simulink model "filtros2"  (R2018b)
settings: Solver=VariableStepAuto  StartTime=0.0  StopTime=10.0  RelTol=1e-3
settings Model: Creator=vini  LastModifiedBy=vini

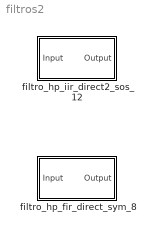
== system filtros2 ==
  filtro_hp_fir_direct_sym_8 : Subsystem  Tag=FilterWizardSubSystem
      settings: ErrorFcn=dspFilterRealizedInBasicElemsAlgLoopErrFcnCallback
  filtro_hp_iir_direct2_sos_12 : Subsystem  Tag=FilterWizardSubSystem
      settings: ErrorFcn=dspFilterRealizedInBasicElemsAlgLoopErrFcnCallback

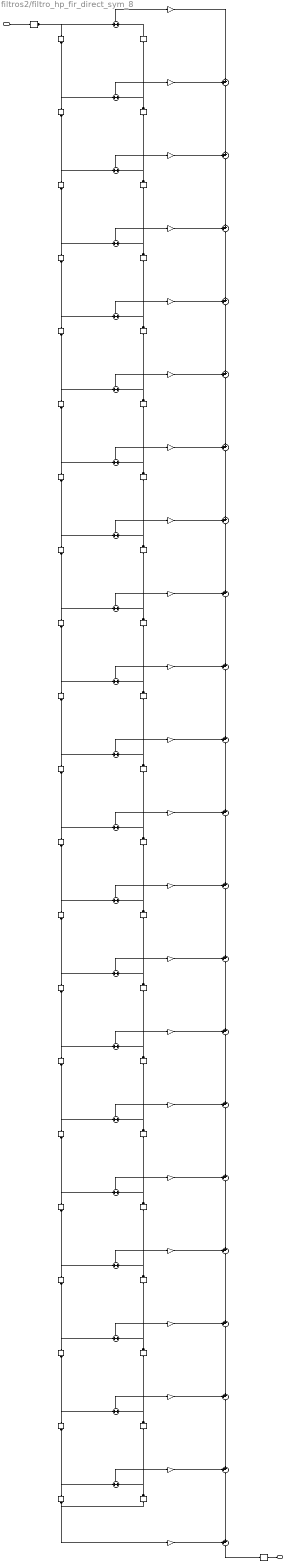
== system filtros2/filtro_hp_fir_direct_sym_8 ==
  Input : Inport
  BodyDelayL{2..21} (20 alike) : Delay  DelayLength=1  InitialCondition=0  InputProcessing=Columns as channels (frame based)
  BodyDelayR{2..21} (20 alike) : Delay  DelayLength=1  InitialCondition=0  InputProcessing=Columns as channels (frame based)
  BodySumL{2..21} (20 alike) : Sum  Inputs=+|+  AccumDataTypeStr=fixdt(1,17,15)  OutDataTypeStr=fixdt(1,17,15)  RndMeth=Convergent
  BodySumR{2..21} (20 alike) : Sum  Inputs=++|  AccumDataTypeStr=fixdt(1,25,23)  OutDataTypeStr=fixdt(1,25,23)  RndMeth=Convergent
  ConvertIn : DataTypeConversion  OutDataTypeStr=fixdt(1,16,15)  RndMeth=Nearest  SaturateOnIntegerOverflow=on
  ConvertOut : DataTypeConversion  OutDataTypeStr=fixdt(1,25,23)  RndMeth=Convergent
  FootDelayL22 : Delay  DelayLength=1  InitialCondition=0  InputProcessing=Columns as channels (frame based)
  FootSumR22 : Sum  Inputs=++|  AccumDataTypeStr=fixdt(1,25,23)  OutDataTypeStr=fixdt(1,25,23)  RndMeth=Convergent
  HeadDelayR1 : Delay  DelayLength=1  InitialCondition=0  InputProcessing=Columns as channels (frame based)
  HeadSumL1 : Sum  Inputs=+|+  AccumDataTypeStr=fixdt(1,17,15)  OutDataTypeStr=fixdt(1,17,15)  RndMeth=Convergent
  h(1) : Gain  Gain=-0.00532709506172761044  ParamDataTypeStr=fixdt(1,8,8)  OutDataTypeStr=fixdt(1,24,23)  RndMeth=Convergent
  h(10) : Gain  Gain=0.00894421000991611065  ParamDataTypeStr=fixdt(1,8,8)  OutDataTypeStr=fixdt(1,24,23)  RndMeth=Convergent
  h(11) : Gain  Gain=-0.0216421575545340458  ParamDataTypeStr=fixdt(1,8,8)  OutDataTypeStr=fixdt(1,24,23)  RndMeth=Convergent
  h(12) : Gain  Gain=0.0030362156599829525  ParamDataTypeStr=fixdt(1,8,8)  OutDataTypeStr=fixdt(1,24,23)  RndMeth=Convergent
  h(13) : Gain  Gain=0.0265962407774834042  ParamDataTypeStr=fixdt(1,8,8)  OutDataTypeStr=fixdt(1,24,23)  RndMeth=Convergent
  h(14) : Gain  Gain=-0.0224925554974460436  ParamDataTypeStr=fixdt(1,8,8)  OutDataTypeStr=fixdt(1,24,23)  RndMeth=Convergent
  h(15) : Gain  Gain=-0.0206671663559229203  ParamDataTypeStr=fixdt(1,8,8)  OutDataTypeStr=fixdt(1,24,23)  RndMeth=Convergent
  h(16) : Gain  Gain=0.0463858207415749138  ParamDataTypeStr=fixdt(1,8,8)  OutDataTypeStr=fixdt(1,24,23)  RndMeth=Convergent
  h(17) : Gain  Gain=-0.00352514866909382297  ParamDataTypeStr=fixdt(1,8,8)  OutDataTypeStr=fixdt(1,24,23)  RndMeth=Convergent
  h(18) : Gain  Gain=-0.0696283973383888116  ParamDataTypeStr=fixdt(1,8,8)  OutDataTypeStr=fixdt(1,24,23)  RndMeth=Convergent
  h(19) : Gain  Gain=0.0620411228742990054  ParamDataTypeStr=fixdt(1,8,8)  OutDataTypeStr=fixdt(1,24,23)  RndMeth=Convergent
  h(2) : Gain  Gain=0.00150016559407488014  ParamDataTypeStr=fixdt(1,8,8)  OutDataTypeStr=fixdt(1,24,23)  RndMeth=Convergent
  h(20) : Gain  Gain=0.0865544797646948944  ParamDataTypeStr=fixdt(1,8,8)  OutDataTypeStr=fixdt(1,24,23)  RndMeth=Convergent
  h(21) : Gain  Gain=-0.292552788167892264  ParamDataTypeStr=fixdt(1,8,8)  OutDataTypeStr=fixdt(1,24,23)  RndMeth=Convergent
  h(22) : Gain  Gain=0.389496680318399457  ParamDataTypeStr=fixdt(1,8,8)  OutDataTypeStr=fixdt(1,24,23)  RndMeth=Convergent
  h(3) : Gain  Gain=0.00628495279823278012  ParamDataTypeStr=fixdt(1,8,8)  OutDataTypeStr=fixdt(1,24,23)  RndMeth=Convergent
  h(4) : Gain  Gain=-0.00636828988327803585  ParamDataTypeStr=fixdt(1,8,8)  OutDataTypeStr=fixdt(1,24,23)  RndMeth=Convergent
  h(5) : Gain  Gain=-0.00403452349221034706  ParamDataTypeStr=fixdt(1,8,8)  OutDataTypeStr=fixdt(1,24,23)  RndMeth=Convergent
  h(6) : Gain  Gain=0.0111906482400220622  ParamDataTypeStr=fixdt(1,8,8)  OutDataTypeStr=fixdt(1,24,23)  RndMeth=Convergent
  h(7) : Gain  Gain=-0.00231967061384724497  ParamDataTypeStr=fixdt(1,8,8)  OutDataTypeStr=fixdt(1,24,23)  RndMeth=Convergent
  h(8) : Gain  Gain=-0.0130613282623932899  ParamDataTypeStr=fixdt(1,8,8)  OutDataTypeStr=fixdt(1,24,23)  RndMeth=Convergent
  h(9) : Gain  Gain=0.01189990154197915  ParamDataTypeStr=fixdt(1,8,8)  OutDataTypeStr=fixdt(1,24,23)  RndMeth=Convergent
  Output : Outport
  wires:
  Input/1 -> ConvertIn/1
  HeadSumL1/1 -> h(1)/1
  h(1)/1 -> BodySumR2/2
  HeadDelayR1/1 -> HeadSumL1/2
  ConvertIn/1 -> HeadSumL1/1, BodyDelayL2/1
  BodyDelayL2/1 -> BodySumL2/1, BodyDelayL3/1
  BodySumL2/1 -> h(2)/1
  h(2)/1 -> BodySumR2/1
  BodyDelayR2/1 -> BodySumL2/2, HeadDelayR1/1
  BodySumR2/1 -> BodySumR3/2
  BodyDelayL3/1 -> BodySumL3/1, BodyDelayL4/1
  BodySumL3/1 -> h(3)/1
  h(3)/1 -> BodySumR3/1
  BodyDelayR3/1 -> BodySumL3/2, BodyDelayR2/1
  BodySumR3/1 -> BodySumR4/2
  BodyDelayL4/1 -> BodySumL4/1, BodyDelayL5/1
  BodySumL4/1 -> h(4)/1
  h(4)/1 -> BodySumR4/1
  BodyDelayR4/1 -> BodySumL4/2, BodyDelayR3/1
  BodySumR4/1 -> BodySumR5/2
  BodyDelayL5/1 -> BodySumL5/1, BodyDelayL6/1
  BodySumL5/1 -> h(5)/1
  h(5)/1 -> BodySumR5/1
  BodyDelayR5/1 -> BodySumL5/2, BodyDelayR4/1
  BodySumR5/1 -> BodySumR6/2
  BodyDelayL6/1 -> BodySumL6/1, BodyDelayL7/1
  BodySumL6/1 -> h(6)/1
  h(6)/1 -> BodySumR6/1
  BodyDelayR6/1 -> BodySumL6/2, BodyDelayR5/1
  BodySumR6/1 -> BodySumR7/2
  BodyDelayL7/1 -> BodySumL7/1, BodyDelayL8/1
  BodySumL7/1 -> h(7)/1
  h(7)/1 -> BodySumR7/1
  BodyDelayR7/1 -> BodySumL7/2, BodyDelayR6/1
  BodySumR7/1 -> BodySumR8/2
  BodyDelayL8/1 -> BodySumL8/1, BodyDelayL9/1
  BodySumL8/1 -> h(8)/1
  h(8)/1 -> BodySumR8/1
  BodyDelayR8/1 -> BodySumL8/2, BodyDelayR7/1
  BodySumR8/1 -> BodySumR9/2
  BodyDelayL9/1 -> BodySumL9/1, BodyDelayL10/1
  BodySumL9/1 -> h(9)/1
  h(9)/1 -> BodySumR9/1
  BodyDelayR9/1 -> BodySumL9/2, BodyDelayR8/1
  BodySumR9/1 -> BodySumR10/2
  BodyDelayL10/1 -> BodySumL10/1, BodyDelayL11/1
  BodySumL10/1 -> h(10)/1
  h(10)/1 -> BodySumR10/1
  BodyDelayR10/1 -> BodySumL10/2, BodyDelayR9/1
  BodySumR10/1 -> BodySumR11/2
  BodyDelayL11/1 -> BodySumL11/1, BodyDelayL12/1
  BodySumL11/1 -> h(11)/1
  h(11)/1 -> BodySumR11/1
  BodyDelayR11/1 -> BodySumL11/2, BodyDelayR10/1
  BodySumR11/1 -> BodySumR12/2
  BodyDelayL12/1 -> BodySumL12/1, BodyDelayL13/1
  BodySumL12/1 -> h(12)/1
  h(12)/1 -> BodySumR12/1
  BodyDelayR12/1 -> BodySumL12/2, BodyDelayR11/1
  BodySumR12/1 -> BodySumR13/2
  BodyDelayL13/1 -> BodySumL13/1, BodyDelayL14/1
  BodySumL13/1 -> h(13)/1
  h(13)/1 -> BodySumR13/1
  BodyDelayR13/1 -> BodySumL13/2, BodyDelayR12/1
  BodySumR13/1 -> BodySumR14/2
  BodyDelayL14/1 -> BodySumL14/1, BodyDelayL15/1
  BodySumL14/1 -> h(14)/1
  h(14)/1 -> BodySumR14/1
  BodyDelayR14/1 -> BodySumL14/2, BodyDelayR13/1
  BodySumR14/1 -> BodySumR15/2
  BodyDelayL15/1 -> BodySumL15/1, BodyDelayL16/1
  BodySumL15/1 -> h(15)/1
  h(15)/1 -> BodySumR15/1
  BodyDelayR15/1 -> BodySumL15/2, BodyDelayR14/1
  BodySumR15/1 -> BodySumR16/2
  BodyDelayL16/1 -> BodySumL16/1, BodyDelayL17/1
  BodySumL16/1 -> h(16)/1
  h(16)/1 -> BodySumR16/1
  BodyDelayR16/1 -> BodySumL16/2, BodyDelayR15/1
  BodySumR16/1 -> BodySumR17/2
  BodyDelayL17/1 -> BodySumL17/1, BodyDelayL18/1
  BodySumL17/1 -> h(17)/1
  h(17)/1 -> BodySumR17/1
  BodyDelayR17/1 -> BodySumL17/2, BodyDelayR16/1
  BodySumR17/1 -> BodySumR18/2
  BodyDelayL18/1 -> BodySumL18/1, BodyDelayL19/1
  BodySumL18/1 -> h(18)/1
  h(18)/1 -> BodySumR18/1
  BodyDelayR18/1 -> BodySumL18/2, BodyDelayR17/1
  BodySumR18/1 -> BodySumR19/2
  BodyDelayL19/1 -> BodySumL19/1, BodyDelayL20/1
  BodySumL19/1 -> h(19)/1
  h(19)/1 -> BodySumR19/1
  BodyDelayR19/1 -> BodySumL19/2, BodyDelayR18/1
  BodySumR19/1 -> BodySumR20/2
  BodyDelayL20/1 -> BodySumL20/1, BodyDelayL21/1
  BodySumL20/1 -> h(20)/1
  h(20)/1 -> BodySumR20/1
  BodyDelayR20/1 -> BodySumL20/2, BodyDelayR19/1
  BodySumR20/1 -> BodySumR21/2
  BodyDelayL21/1 -> BodySumL21/1, FootDelayL22/1
  BodySumL21/1 -> h(21)/1
  h(21)/1 -> BodySumR21/1
  BodyDelayR21/1 -> BodySumL21/2, BodyDelayR20/1
  BodySumR21/1 -> FootSumR22/2
  FootDelayL22/1 -> h(22)/1, BodyDelayR21/1
  h(22)/1 -> FootSumR22/1
  FootSumR22/1 -> ConvertOut/1
  ConvertOut/1 -> Output/1

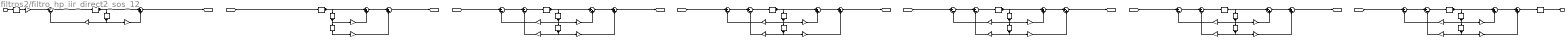
== system filtros2/filtro_hp_iir_direct2_sos_12 ==
  Input : Inport
  CastState{1..7} (7 alike) : DataTypeConversion  OutDataTypeStr=fixdt(1,16,15)  RndMeth=Convergent
  ConvertIn : DataTypeConversion  OutDataTypeStr=fixdt(1,16,15)  RndMeth=Nearest  SaturateOnIntegerOverflow=on
  ConvertOut : DataTypeConversion  OutDataTypeStr=fixdt(1,16,7)  RndMeth=Convergent
  Delay{11..17,22..27} (13 alike) : Delay  DelayLength=1  InitialCondition=0
  SumA{21,23..27,33..37} (11 alike) : Sum  Inputs=|+-  AccumDataTypeStr=fixdt(1,30,25)  OutDataTypeStr=fixdt(1,30,25)  RndMeth=Convergent
  SumB{21..27,32..37} (13 alike) : Sum  Inputs=|++  AccumDataTypeStr=fixdt(1,30,21)  OutDataTypeStr=fixdt(1,30,21)  RndMeth=Convergent
  a(2)(1) : Gain  Gain=0.415474721603748653  ParamDataTypeStr=fixdt(1,12,10)  OutDataTypeStr=fixdt(1,28,25)  RndMeth=Convergent
  a(2)(3) : Gain  Gain=-0.0534464222346326817  ParamDataTypeStr=fixdt(1,12,10)  OutDataTypeStr=fixdt(1,28,25)  RndMeth=Convergent
  a(2)(4) : Gain  Gain=0.912430013497696479  ParamDataTypeStr=fixdt(1,12,10)  OutDataTypeStr=fixdt(1,28,25)  RndMeth=Convergent
  a(2)(5) : Gain  Gain=0.700912460681827776  ParamDataTypeStr=fixdt(1,12,10)  OutDataTypeStr=fixdt(1,28,25)  RndMeth=Convergent
  a(2)(6) : Gain  Gain=0.336705133533832024  ParamDataTypeStr=fixdt(1,12,10)  OutDataTypeStr=fixdt(1,28,25)  RndMeth=Convergent
  a(2)(7) : Gain  Gain=0.672299092917526986  ParamDataTypeStr=fixdt(1,12,10)  OutDataTypeStr=fixdt(1,28,25)  RndMeth=Convergent
  a(3)(3) : Gain  Gain=0.155789387270914625  ParamDataTypeStr=fixdt(1,12,10)  OutDataTypeStr=fixdt(1,28,25)  RndMeth=Convergent
  a(3)(4) : Gain  Gain=0.311516679849097922  ParamDataTypeStr=fixdt(1,12,10)  OutDataTypeStr=fixdt(1,28,25)  RndMeth=Convergent
  a(3)(5) : Gain  Gain=0.455486580885583192  ParamDataTypeStr=fixdt(1,12,10)  OutDataTypeStr=fixdt(1,28,25)  RndMeth=Convergent
  a(3)(6) : Gain  Gain=0.516670640463280928  ParamDataTypeStr=fixdt(1,12,10)  OutDataTypeStr=fixdt(1,28,25)  RndMeth=Convergent
  a(3)(7) : Gain  Gain=0.823202885567432596  ParamDataTypeStr=fixdt(1,12,10)  OutDataTypeStr=fixdt(1,28,25)  RndMeth=Convergent
  b(2)(1) : Gain  Gain=-0.99999999999989253  ParamDataTypeStr=fixdt(1,12,6)  OutDataTypeStr=fixdt(1,28,21)  RndMeth=Convergent
  b(2)(2) : Gain  Gain=-8.07609406410542263  ParamDataTypeStr=fixdt(1,12,6)  OutDataTypeStr=fixdt(1,28,21)  RndMeth=Convergent
  b(2)(3) : Gain  Gain=-1.53376334450087937  ParamDataTypeStr=fixdt(1,12,6)  OutDataTypeStr=fixdt(1,28,21)  RndMeth=Convergent
  b(2)(4) : Gain  Gain=-1.6085731579110969  ParamDataTypeStr=fixdt(1,12,6)  OutDataTypeStr=fixdt(1,28,21)  RndMeth=Convergent
  b(2)(5) : Gain  Gain=-0.414584614039461674  ParamDataTypeStr=fixdt(1,12,6)  OutDataTypeStr=fixdt(1,28,21)  RndMeth=Convergent
  b(2)(6) : Gain  Gain=-0.910081099356177647  ParamDataTypeStr=fixdt(1,12,6)  OutDataTypeStr=fixdt(1,28,21)  RndMeth=Convergent
  b(2)(7) : Gain  Gain=-0.456903720087069476  ParamDataTypeStr=fixdt(1,12,6)  OutDataTypeStr=fixdt(1,28,21)  RndMeth=Convergent
  b(3)(2) : Gain  Gain=19.479965706920094  ParamDataTypeStr=fixdt(1,12,6)  OutDataTypeStr=fixdt(1,28,21)  RndMeth=Convergent
  b(3)(3) : Gain  Gain=3.35686333262635195  ParamDataTypeStr=fixdt(1,12,6)  OutDataTypeStr=fixdt(1,28,21)  RndMeth=Convergent
  b(3)(4) : Gain  Gain=1.00000000000014611  ParamDataTypeStr=fixdt(1,12,6)  OutDataTypeStr=fixdt(1,28,21)  RndMeth=Convergent
  b(3)(5) : Gain  Gain=0.0513347926297817794  ParamDataTypeStr=fixdt(1,12,6)  OutDataTypeStr=fixdt(1,28,21)  RndMeth=Convergent
  b(3)(6) : Gain  Gain=0.999999999999969691  ParamDataTypeStr=fixdt(1,12,6)  OutDataTypeStr=fixdt(1,28,21)  RndMeth=Convergent
  b(3)(7) : Gain  Gain=0.297897144122819202  ParamDataTypeStr=fixdt(1,12,6)  OutDataTypeStr=fixdt(1,28,21)  RndMeth=Convergent
  s(1) : Gain  Gain=3.0517578125e-05  ParamDataTypeStr=fixdt(1,12,25)  OutDataTypeStr=fixdt(1,16,20)  RndMeth=Convergent
  Output : Outport
  wires:
  Input/1 -> ConvertIn/1
  s(1)/1 -> SumA21/1
  SumA21/1 -> CastState1/1
  CastState1/1 -> SumB21/1, Delay11/1
  SumB21/1 -> [Sect1]
  a(2)(1)/1 -> SumA21/2
  Delay11/1 -> a(2)(1)/1, b(2)(1)/1
  b(2)(1)/1 -> SumB21/2
  ConvertIn/1 -> s(1)/1
  [Sect1] -> CastState2/1
  CastState2/1 -> SumB22/1, Delay12/1
  SumB22/1 -> SumB32/1
  SumB32/1 -> [Sect2]
  Delay12/1 -> b(2)(2)/1, Delay22/1
  b(2)(2)/1 -> SumB22/2
  Delay22/1 -> b(3)(2)/1
  b(3)(2)/1 -> SumB32/2
  [Sect2] -> SumA23/1
  SumA23/1 -> SumA33/1
  SumA33/1 -> CastState3/1
  CastState3/1 -> SumB23/1, Delay13/1
  SumB23/1 -> SumB33/1
  SumB33/1 -> [Sect3]
  a(2)(3)/1 -> SumA23/2
  Delay13/1 -> a(2)(3)/1, b(2)(3)/1, Delay23/1
  b(2)(3)/1 -> SumB23/2
  a(3)(3)/1 -> SumA33/2
  Delay23/1 -> a(3)(3)/1, b(3)(3)/1
  b(3)(3)/1 -> SumB33/2
  [Sect3] -> SumA24/1
  SumA24/1 -> SumA34/1
  SumA34/1 -> CastState4/1
  CastState4/1 -> SumB24/1, Delay14/1
  SumB24/1 -> SumB34/1
  SumB34/1 -> [Sect4]
  a(2)(4)/1 -> SumA24/2
  Delay14/1 -> a(2)(4)/1, b(2)(4)/1, Delay24/1
  b(2)(4)/1 -> SumB24/2
  a(3)(4)/1 -> SumA34/2
  Delay24/1 -> a(3)(4)/1, b(3)(4)/1
  b(3)(4)/1 -> SumB34/2
  [Sect4] -> SumA25/1
  SumA25/1 -> SumA35/1
  SumA35/1 -> CastState5/1
  CastState5/1 -> SumB25/1, Delay15/1
  SumB25/1 -> SumB35/1
  SumB35/1 -> [Sect5]
  a(2)(5)/1 -> SumA25/2
  Delay15/1 -> a(2)(5)/1, b(2)(5)/1, Delay25/1
  b(2)(5)/1 -> SumB25/2
  a(3)(5)/1 -> SumA35/2
  Delay25/1 -> a(3)(5)/1, b(3)(5)/1
  b(3)(5)/1 -> SumB35/2
  [Sect5] -> SumA26/1
  SumA26/1 -> SumA36/1
  SumA36/1 -> CastState6/1
  CastState6/1 -> SumB26/1, Delay16/1
  SumB26/1 -> SumB36/1
  SumB36/1 -> [Sect6]
  a(2)(6)/1 -> SumA26/2
  Delay16/1 -> a(2)(6)/1, b(2)(6)/1, Delay26/1
  b(2)(6)/1 -> SumB26/2
  a(3)(6)/1 -> SumA36/2
  Delay26/1 -> a(3)(6)/1, b(3)(6)/1
  b(3)(6)/1 -> SumB36/2
  [Sect6] -> SumA27/1
  SumA27/1 -> SumA37/1
  SumA37/1 -> CastState7/1
  CastState7/1 -> SumB27/1, Delay17/1
  SumB27/1 -> SumB37/1
  SumB37/1 -> ConvertOut/1
  a(2)(7)/1 -> SumA27/2
  Delay17/1 -> a(2)(7)/1, b(2)(7)/1, Delay27/1
  b(2)(7)/1 -> SumB27/2
  a(3)(7)/1 -> SumA37/2
  Delay27/1 -> a(3)(7)/1, b(3)(7)/1
  b(3)(7)/1 -> SumB37/2
  ConvertOut/1 -> Output/1
